simulink model "Bloco_SC_CC_PMDC_Chopper"  (R2021a)
settings: Solver=ode4  StartTime=0  StopTime=0.2  FixedStep=1e-8  RelTol=1e-3
values from neighbouring files (symbols this model uses):
  B = 0    [P1_script.m]    (also in simulacao1.m)
  Ia_rated = 25    [P1_script.m]    (also in simulacao1.m)
  J = 0.001    [P1_script.m]    (also in simulacao1.m = 0.00252)
  Kac = 1/Kpc    (= 0.0936205547599)    [P1_script.m]
  Kas = 1/Kps    (= 0.676014937262)    [P1_script.m]
  Kic = Ra*2*pi*Wcc    (= 1633.62817987)    [P1_script.m]
  Kis = J*(2*pi*Wcs)^2/(5*Kt)    (= 185.888948923)    [P1_script.m]
  Kpc = La*2*pi*Wcc    (= 10.6814150222)    [P1_script.m]
  Kps = J*2*pi*Wcs/Kt    (= 1.47925725436)    [P1_script.m]
  Kt = Te_rated/Ia_rated    (= 0.424752712124)    [P1_script.m]    (also in simulacao1.m)
  La = 1.7e-3    (= 0.0017)    [P1_script.m]    (also in simulacao1.m)
  Ra = 0.26    [P1_script.m]    (also in simulacao1.m)
  Te_rated = Power/Wm_rated    (= 10.6188178031)    [P1_script.m]    (also in simulacao1.m)
  Va_rated = 140    [P1_script.m]    (also in simulacao1.m)
  Vdc = Va_rated    (= 140)    [P1_script.m]
libraries: simulink x2
settings Model: Creator=taylo  LastModifiedBy=taylo

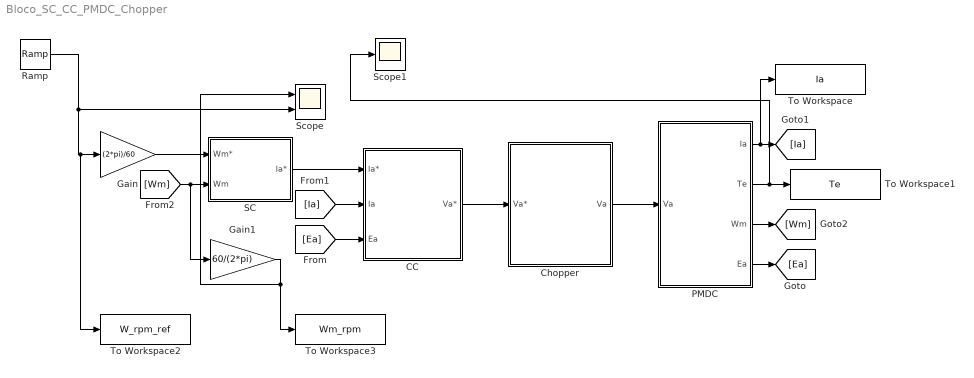
== system Bloco_SC_CC_PMDC_Chopper ==
  CC : Subsystem
  Chopper : Subsystem
  Gain : Gain  Gain=(2*pi)/60
  Gain1 : Gain  Gain=60/(2*pi)
  PMDC : Subsystem
  Ramp : simulink/Sources/Ramp  slope=50  start=0.05  InitialOutput=0
  SC : Subsystem
  Scope : Scope  NumInputPorts=2
  Scope1 : Scope
  To Workspace : ToWorkspace  VariableName=Ia  SaveFormat=Timeseries  SampleTime=-1
  To Workspace1 : ToWorkspace  VariableName=Te  SaveFormat=Timeseries  SampleTime=-1
  To Workspace2 : ToWorkspace  VariableName=W_rpm_ref  SaveFormat=Timeseries  SampleTime=-1
  To Workspace3 : ToWorkspace  VariableName=Wm_rpm  SaveFormat=Timeseries  SampleTime=-1
  wires:
  Gain/1 -> SC/1(Wm*)
  SC/1(Ia*) -> CC/1(Ia*)
  CC/1(Va*) -> Chopper/1(Va*)
  Chopper/1(Va) -> PMDC/1(Va)
  PMDC/1(Ia) -> To Workspace/1, [Ia]
  PMDC/3(Wm) -> [Wm]
  [Wm] -> Gain1/1, SC/2(Wm)
  [Ia] -> CC/2(Ia)
  [Ea] -> CC/3(Ea)
  PMDC/4(Ea) -> [Ea]
  PMDC/2(Te) -> Scope1/1, To Workspace1/1
  Gain1/1 -> Scope/1, To Workspace3/1
  Ramp/1 -> Scope/2, To Workspace2/1, Gain/1

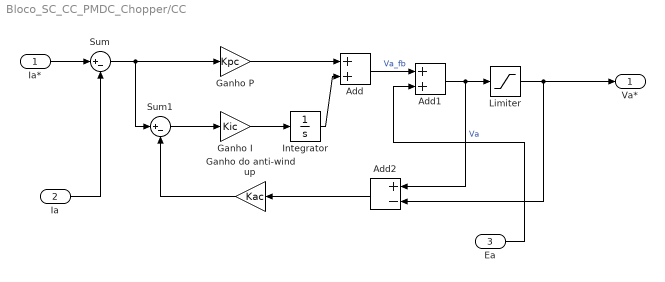
== system Bloco_SC_CC_PMDC_Chopper/CC ==
  Ia* : Inport
  Ia : Inport  Port=2
  Ea : Inport  Port=3
  Add : Sum
  Add1 : Sum
  Add2 : Sum  Inputs=+-
  Ganho I : Gain  Gain=Kic
  Ganho P : Gain  Gain=Kpc
  Ganho do anti-wind up : Gain  Gain=Kac
  Integrator : Integrator
  Limiter : Saturate  UpperLimit=Va_rated  LowerLimit=-Va_rated
  Sum : Sum  Inputs=|+-
  Sum1 : Sum  Inputs=|+-
  Va* : Outport
  wires:
  Ea/1 -> Add1/2
  Limiter/1 -> Va*/1, Add2/2
  Sum/1 -> Sum1/1, Ganho P/1
  Sum1/1 -> Ganho I/1
  Add1/1 -> Add2/1, Limiter/1  "Va"
  Ganho P/1 -> Add/1
  Add/1 -> Add1/1  "Va_fb"
  Ganho I/1 -> Integrator/1
  Integrator/1 -> Add/2
  Ganho do anti-wind up/1 -> Sum1/2
  Add2/1 -> Ganho do anti-wind up/1
  Ia*/1 -> Sum/1
  Ia/1 -> Sum/2

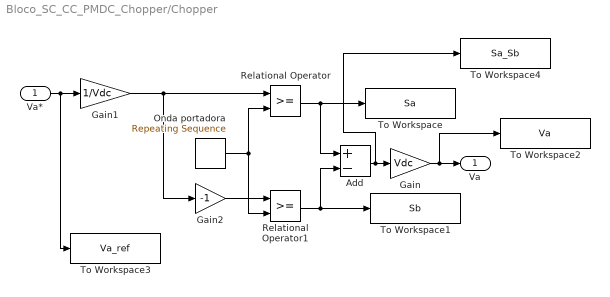
== system Bloco_SC_CC_PMDC_Chopper/Chopper ==
  Va* : Inport
  Add : Sum  Inputs=+-
  Gain : Gain  Gain=Vdc
  Gain1 : Gain  Gain=1/Vdc
  Gain2 : Gain  Gain=-1
  Onda portadora : simulink/Sources/Repeating Sequence  rep_seq_t=[0 1/10000 1/5000]  rep_seq_y=[-1 1 -1]
  Relational Operator : RelationalOperator  OutDataTypeStr=boolean  RndMeth=Simplest
  Relational Operator1 : RelationalOperator  OutDataTypeStr=boolean  RndMeth=Simplest
  To Workspace : ToWorkspace  VariableName=Sa  SaveFormat=Timeseries  SampleTime=-1
  To Workspace1 : ToWorkspace  VariableName=Sb  SaveFormat=Timeseries  SampleTime=-1
  To Workspace2 : ToWorkspace  VariableName=Va  SaveFormat=Timeseries  SampleTime=-1
  To Workspace3 : ToWorkspace  VariableName=Va_ref  SaveFormat=Timeseries  SampleTime=-1
  To Workspace4 : ToWorkspace  VariableName=Sa_Sb  SaveFormat=Timeseries  SampleTime=-1
  Va : Outport
  wires:
  Gain1/1 -> Relational Operator/1, Gain2/1
  Va*/1 -> To Workspace3/1, Gain1/1
  Onda portadora/1 -> Relational Operator1/2, Relational Operator/2
  Gain2/1 -> Relational Operator1/1
  Relational Operator/1 -> To Workspace/1, Add/1
  Relational Operator1/1 -> To Workspace1/1, Add/2
  Add/1 -> To Workspace4/1, Gain/1
  Gain/1 -> To Workspace2/1, Va/1

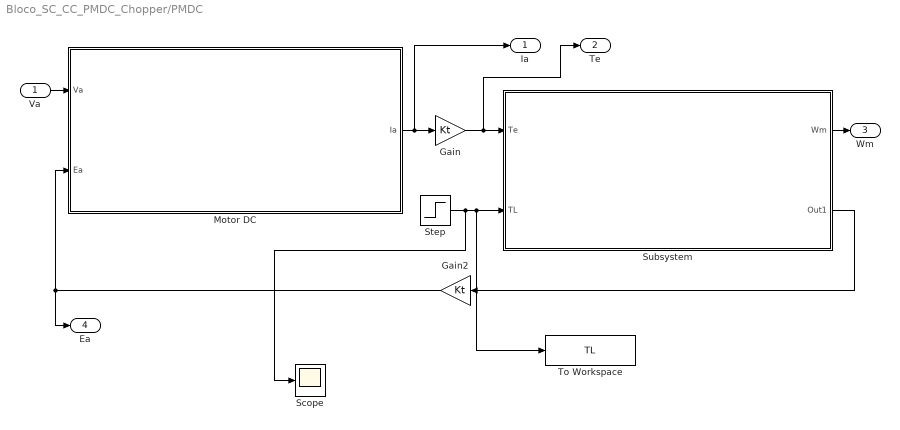
== system Bloco_SC_CC_PMDC_Chopper/PMDC ==
  Va : Inport
  Gain : Gain  Gain=Kt
  Gain2 : Gain  Gain=Kt
  Motor DC : Subsystem
  Scope : Scope
  Step : Step  Time=0.01  After=4  SampleTime=0
  Subsystem : Subsystem
  To Workspace : ToWorkspace  VariableName=TL  SaveFormat=Timeseries  SampleTime=-1
  Ia : Outport
  Te : Outport  Port=2
  Wm : Outport  Port=3
  Ea : Outport  Port=4
  wires:
  Gain/1 -> Te/1, Subsystem/1(Te)
  Step/1 -> Scope/1, To Workspace/1, Subsystem/2(TL)
  Subsystem/2(Out1) -> Gain2/1
  Gain2/1 -> Motor DC/2(Ea), Ea/1
  Motor DC/1(Ia) -> Ia/1, Gain/1
  Subsystem/1(Wm) -> Wm/1
  Va/1 -> Motor DC/1(Va)

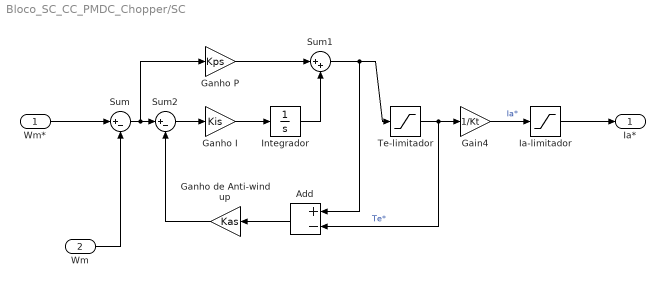
== system Bloco_SC_CC_PMDC_Chopper/SC ==
  Wm* : Inport
  Wm : Inport  Port=2
  Add : Sum  Inputs=+-
  Gain4 : Gain  Gain=1/Kt
  Ganho I : Gain  Gain=Kis
  Ganho P : Gain  Gain=Kps
  Ganho de Anti-wind up : Gain  Gain=Kas
  Ia-limitador : Saturate  UpperLimit=Ia_rated  LowerLimit=-Ia_rated
  Integrador : Integrator
  Sum : Sum  Inputs=|+-
  Sum1 : Sum  Inputs=|++
  Sum2 : Sum  Inputs=|+-
  Te-limitador : Saturate  UpperLimit=Te_rated  LowerLimit=-Te_rated
  Ia* : Outport
  wires:
  Ganho P/1 -> Sum1/1
  Sum1/1 -> Add/1, Te-limitador/1
  Ganho I/1 -> Integrador/1
  Te-limitador/1 -> Add/2, Gain4/1  "Te*"
  Integrador/1 -> Sum1/2
  Sum/1 -> Ganho P/1, Sum2/1
  Wm/1 -> Sum/2
  Ganho de Anti-wind up/1 -> Sum2/2
  Ia-limitador/1 -> Ia*/1
  Gain4/1 -> Ia-limitador/1  "Ia*"
  Sum2/1 -> Ganho I/1
  Add/1 -> Ganho de Anti-wind up/1
  Wm*/1 -> Sum/1

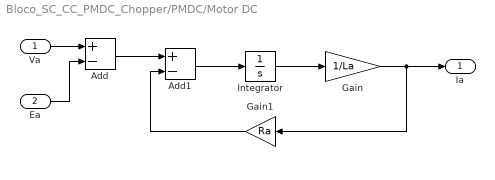
== system Bloco_SC_CC_PMDC_Chopper/PMDC/Motor DC ==
  Va : Inport
  Ea : Inport  Port=2
  Add : Sum  Inputs=+-
  Add1 : Sum  Inputs=+-
  Gain : Gain  Gain=1/La
  Gain1 : Gain  Gain=Ra
  Integrator : Integrator
  Ia : Outport
  wires:
  Add1/1 -> Integrator/1
  Gain1/1 -> Add1/2
  Add/1 -> Add1/1
  Va/1 -> Add/1
  Integrator/1 -> Gain/1
  Ea/1 -> Add/2
  Gain/1 -> Gain1/1, Ia/1

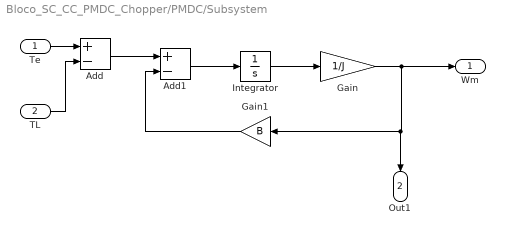
== system Bloco_SC_CC_PMDC_Chopper/PMDC/Subsystem ==
  Te : Inport
  TL : Inport  Port=2
  Add : Sum  Inputs=+-
  Add1 : Sum  Inputs=+-
  Gain : Gain  Gain=1/J
  Gain1 : Gain  Gain=B
  Integrator : Integrator
  Wm : Outport
  Out1 : Outport  Port=2
  wires:
  Te/1 -> Add/1
  Gain/1 -> Wm/1, Out1/1, Gain1/1
  Add/1 -> Add1/1
  TL/1 -> Add/2
  Add1/1 -> Integrator/1
  Gain1/1 -> Add1/2
  Integrator/1 -> Gain/1
